simulink model "sampleModel1607_3_sub"  (R2023a)
settings: Solver=VariableStepAuto  StartTime=0.0  StopTime=10.0  RelTol=1e-3
libraries: hdlsllib x2, simulink x1
settings Model: Creator=user1  LastModifiedBy=user1

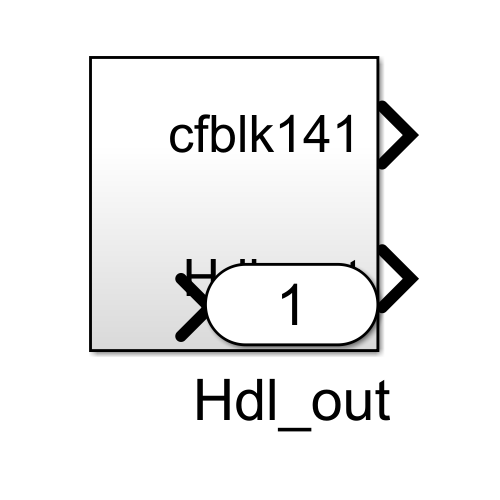
[thumbnail: Simulink's stored preview of the top-level diagram]
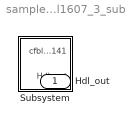
== system sampleModel1607_3_sub ==
  Subsystem : Subsystem
  Hdl_out : Outport  OutDataTypeStr=uint8

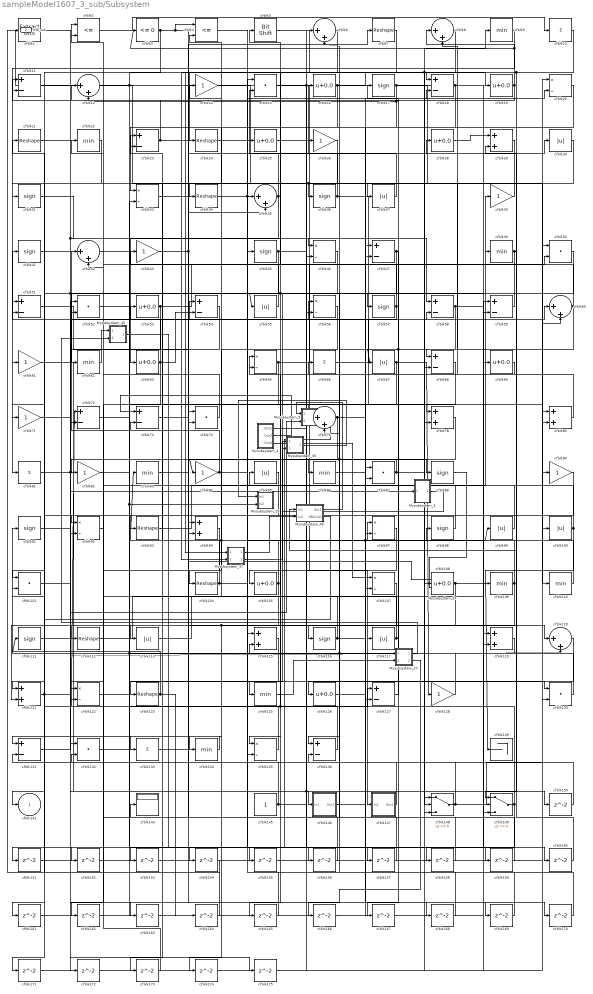
== system sampleModel1607_3_sub/Subsystem ==
  Mysubsystem_19 : Subsystem  TreatAsAtomicUnit=on  RTWFcnName=Mysubsystem_19
      settings: RTWFcnNameOpts=User specified  RTWFileNameOpts=Use function name
  Mysubsystem_2 : Subsystem  TreatAsAtomicUnit=on  RTWFcnName=Mysubsystem_2
      settings: RTWFcnNameOpts=User specified  RTWFileNameOpts=Use function name
  Mysubsystem_24 : Subsystem  TreatAsAtomicUnit=on  RTWFcnName=Mysubsystem_24
      settings: RTWFcnNameOpts=User specified  RTWFileNameOpts=Use function name
  Mysubsystem_27 : Subsystem  TreatAsAtomicUnit=on  RTWFcnName=Mysubsystem_27
      settings: RTWFcnNameOpts=User specified  RTWFileNameOpts=Use function name
  Mysubsystem_3 : Subsystem  TreatAsAtomicUnit=on  RTWFcnName=Mysubsystem_3
      settings: RTWFcnNameOpts=User specified  RTWFileNameOpts=Use function name
  Mysubsystem_35 : Subsystem  TreatAsAtomicUnit=on  RTWFcnName=Mysubsystem_35
      settings: RTWFcnNameOpts=User specified  RTWFileNameOpts=Use function name
  Mysubsystem_37 : Subsystem  TreatAsAtomicUnit=on  RTWFcnName=Mysubsystem_37
      settings: RTWFcnNameOpts=User specified  RTWFileNameOpts=Use function name
  Mysubsystem_43 : Subsystem  TreatAsAtomicUnit=on  RTWFcnName=Mysubsystem_43
      settings: RTWFcnNameOpts=User specified  RTWFileNameOpts=Use function name
  Mysubsystem_45 : Subsystem  TreatAsAtomicUnit=on  RTWFcnName=Mysubsystem_45
      settings: RTWFcnNameOpts=User specified  RTWFileNameOpts=Use function name
  Mysubsystem_5 : Subsystem  TreatAsAtomicUnit=on  RTWFcnName=Mysubsystem_5
      settings: RTWFcnNameOpts=User specified  RTWFileNameOpts=Use function name
  cfblk1 : simulink/Logic and Bit Operations/Extract Bits  bitsToExtract=Upper half  numBits=8  bitIdxRange=[0 7]  outScalingMode=Preserve fixed-point scaling
      settings: LibrarySourceBlock=|
      | hdlsllib/Logic and Bit
      | Operations/Extract Bits
  cfblk{10,66,81,133} (4 alike) : Sum  Inputs=+  OutDataTypeStr=uint8
  cfblk{30,37,55,67,85,99..100,113,117} (9 alike) : Abs  OutDataTypeStr=uint8  SaturateOnIntegerOverflow=off
  cfblk{15,50,52,74,87,101,130,132} (8 alike) : DotProduct  OutDataTypeStr=uint8
  cfblk{7,21,24,34,93,104,112,123} (8 alike) : Reshape
  cfblk{16,19,25,28,53,63,69,105,108,126} (10 alike) : Bias  Bias=0.0  SaturateOnIntegerOverflow=off
  cfblk{20,33,46,56,65,92,97,107,122,135} (10 alike) : Product  Inputs=*/  OutDataTypeStr=uint8  RndMeth=Zero  SaturateOnIntegerOverflow=on
  cfblk{9,22,49,62,83,86,109..110,125,134} (10 alike) : MinMax  OutDataTypeStr=uint8
  cfblk{11,18,23,47,51,54,58..59,68,72..73,127,131,136} (14 alike) : Sum  Inputs=+-  OutDataTypeStr=uint8
  cfblk{17,31,36,41,45,57,88,91,98,111,116} (11 alike) : Signum
  cfblk{29,78,80,94,115,119,121} (7 alike) : Sum  OutDataTypeStr=uint8
  cfblk{6,8,12,35,42,60,76,120} (8 alike) : Sum  Inputs=|++  OutDataTypeStr=uint8
  cfblk{14,26,39,43,61,71,82,84,90,128} (10 alike) : Gain  OutDataTypeStr=uint8
  cfblk139 : Terminator
  cfblk143 : Display
  cfblk145 : Constant  OutDataTypeStr=uint8  SampleTime=-1
  cfblk146 : Subsystem
      settings: LibrarySourceBlock=|
      | hdlsllib/Ports &
      | Subsystems/Subsystem
  cfblk147 : Subsystem
      settings: LibrarySourceBlock=|
      | hdlsllib/Ports &
      | Subsystems/Subsystem
  cfblk148 : Switch  OutDataTypeStr=uint8  SaturateOnIntegerOverflow=off  InputSameDT=off
  cfblk149 : Switch  OutDataTypeStr=uint8  SaturateOnIntegerOverflow=off  InputSameDT=off
  cfblk{150..175} (26 alike) : Delay  SampleTime=1
  cfblk2 : RelationalOperator  Operator=<=  OutDataTypeStr=boolean  InputSameDT=off
  cfblk3 : hdlsllib/Logic and Bit Operations/Compare To Zero  relop=<=  OutDataTypeStr=uint8
  cfblk4 : RelationalOperator  Operator=<=  OutDataTypeStr=boolean  InputSameDT=off
  cfblk5 : hdlsllib/Logic and Bit Operations/Bit Shift  mode=Shift Left Logical  N=0
  cfblk141 : Outport  OutDataTypeStr=uint8  VectorParamsAs1DForOutWhenUnconnected=off
  Hdl_out : Outport  Port=2  OutDataTypeStr=uint8
  wires:
  cfblk10/1 -> cfblk149/1, cfblk68/2, Mysubsystem_37/2(In2)
  cfblk9/1 -> cfblk81/1
  cfblk47/1 -> cfblk123/1, cfblk167/1, cfblk67/1
  cfblk35/1 -> cfblk15/2, cfblk63/1
  cfblk6/1 -> cfblk165/1, cfblk55/1
  cfblk61/1 -> cfblk146/1(In1)
  cfblk84/1 -> cfblk18/2, cfblk42/1
  cfblk2/1 -> cfblk10/1
  cfblk136/1 -> cfblk85/1, cfblk72/1
  cfblk120/1 -> cfblk143/1
  cfblk78/1 -> cfblk116/1, cfblk84/1
  cfblk108/1 -> cfblk121/2, cfblk139/1
  cfblk110/1 -> cfblk54/1, cfblk83/1
  cfblk24/1 -> cfblk100/1
  cfblk93/1 -> cfblk39/1
  cfblk97/1 -> cfblk135/1
  cfblk41/1 -> cfblk132/1
  cfblk67/1 -> cfblk125/1, cfblk128/1
  cfblk15/1 -> cfblk107/2, cfblk147/1(In1)
  cfblk99/1 -> cfblk65/1
  cfblk3/1 -> cfblk71/1, cfblk120/1, cfblk4/1
  cfblk31/1 -> cfblk46/1
  cfblk60/1 -> cfblk23/1, cfblk126/1
  cfblk107/1 -> cfblk174/1, cfblk133/1
  cfblk65/1 -> cfblk113/1, cfblk49/1
  cfblk26/1 -> cfblk93/1
  cfblk55/1 -> cfblk22/1
  cfblk149/1 -> cfblk171/1, cfblk66/1
  cfblk21/1 -> cfblk46/2
  cfblk22/1 -> cfblk61/1
  cfblk123/1 -> cfblk164/1, cfblk91/1
  cfblk36/1 -> cfblk25/1, cfblk110/1
  cfblk117/1 -> cfblk157/1, cfblk4/2
  cfblk39/1 -> cfblk31/1
  cfblk130/1 -> cfblk17/1
  cfblk57/1 -> cfblk51/2, cfblk5/1
  cfblk109/1 -> cfblk162/1, cfblk43/1
  cfblk104/1 -> cfblk98/1, cfblk73/2
  cfblk82/1 -> cfblk56/1
  cfblk49/1 -> cfblk117/1, Mysubsystem_43/1(In1)
  cfblk132/1 -> cfblk127/1
  cfblk20/1 -> cfblk105/1
  cfblk68/1 -> cfblk135/2
  cfblk98/1 -> cfblk2/1
  cfblk94/1 -> cfblk112/1
  cfblk8/1 -> cfblk24/1
  cfblk135/1 -> cfblk21/1
  cfblk134/1 -> cfblk131/1
  cfblk105/1 -> cfblk173/1, cfblk14/1
  cfblk119/1 -> cfblk115/2
  cfblk17/1 -> cfblk60/2, cfblk12/2, cfblk33/1
  cfblk37/1 -> cfblk16/1
  cfblk14/1 -> cfblk37/1
  cfblk126/1 -> cfblk20/2, cfblk99/1
  cfblk76/1 -> cfblk94/2, cfblk30/1
  cfblk127/1 -> cfblk97/1
  cfblk128/1 -> cfblk6/2, cfblk111/1
  cfblk28/1 -> cfblk29/1
  cfblk42/1 -> cfblk130/1, Mysubsystem_19/2(In2)
  cfblk116/1 -> cfblk149/3, cfblk2/2
  cfblk18/1 -> Hdl_out/1, cfblk87/2, cfblk119/1
  cfblk19/1 -> cfblk11/2, cfblk3/1, cfblk8/1
  cfblk63/1 -> cfblk54/2, cfblk92/1, cfblk41/1
  cfblk5/1 -> cfblk148/2
  cfblk121/1 -> cfblk151/1, cfblk150/1
  cfblk59/1 -> cfblk57/1
  cfblk80/1 -> cfblk8/2
  cfblk100/1 -> cfblk23/2, cfblk109/1
  cfblk16/1 -> cfblk19/1, cfblk34/1
  cfblk46/1 -> cfblk121/1
  cfblk72/1 -> cfblk78/1
  cfblk56/1 -> cfblk104/1
  cfblk33/1 -> cfblk35/2
  cfblk25/1 -> cfblk58/1
  cfblk147/1(Out1) -> cfblk51/1
  cfblk45/1 -> cfblk159/1, cfblk62/1
  cfblk131/1 -> cfblk52/1
  cfblk90/1 -> cfblk122/1
  cfblk51/1 -> cfblk74/2
  cfblk87/1 -> cfblk9/1, cfblk82/1
  cfblk122/1 -> Mysubsystem_27/1(In1), cfblk50/2
  cfblk1/1 -> cfblk120/2, cfblk59/2
  cfblk12/1 -> cfblk154/1, cfblk18/1, cfblk108/1
  cfblk113/1 -> cfblk45/1
  cfblk69/1 -> cfblk65/2
  cfblk85/1 -> cfblk101/1
  cfblk74/1 -> cfblk12/1
  cfblk58/1 -> cfblk160/1, cfblk76/1
  cfblk53/1 -> cfblk92/2, cfblk20/1
  cfblk50/1 -> cfblk136/1
  cfblk23/1 -> cfblk169/1, cfblk11/1
  cfblk11/1 -> cfblk168/1, cfblk47/2
  cfblk73/1 -> cfblk86/1
  cfblk112/1 -> cfblk69/1
  cfblk83/1 -> cfblk7/1
  cfblk115/1 -> cfblk134/1
  cfblk66/1 -> cfblk58/2
  cfblk81/1 -> cfblk53/1, Mysubsystem_3/1(In1)
  cfblk146/1(Out1) -> cfblk97/2
  cfblk52/1 -> cfblk80/2
  cfblk148/1 -> cfblk52/2, cfblk90/1
  cfblk34/1 -> cfblk26/1, cfblk88/1
  cfblk30/1 -> cfblk68/1
  cfblk133/1 -> cfblk94/1
  cfblk29/1 -> cfblk161/1, cfblk36/1
  cfblk43/1 -> cfblk28/1, Mysubsystem_24/1(In1)
  cfblk145/1 -> cfblk101/2, cfblk149/2, cfblk60/1
  cfblk150/1 -> cfblk132/2
  cfblk151/1 -> cfblk127/2
  cfblk92/1 -> cfblk152/1
  cfblk152/1 -> cfblk35/1
  cfblk54/1 -> cfblk153/1
  cfblk153/1 -> cfblk50/1
  cfblk154/1 -> cfblk1/1
  cfblk155/1 -> cfblk80/1
  cfblk4/1 -> cfblk156/1
  cfblk156/1 -> cfblk42/2
  cfblk157/1 -> cfblk122/2
  cfblk158/1 -> cfblk74/1
  cfblk159/1 -> cfblk76/2
  cfblk160/1 -> cfblk29/2
  cfblk161/1 -> cfblk78/2
  cfblk162/1 -> cfblk33/2
  cfblk91/1 -> cfblk163/1
  cfblk163/1 -> cfblk119/2
  cfblk164/1 -> cfblk131/2
  cfblk165/1 -> cfblk115/1
  cfblk166/1 -> cfblk47/1
  cfblk167/1 -> cfblk148/3
  cfblk168/1 -> cfblk15/1
  cfblk169/1 -> cfblk136/2
  cfblk86/1 -> cfblk170/1
  cfblk170/1 -> cfblk87/1
  cfblk171/1 -> cfblk56/2
  cfblk71/1 -> cfblk172/1
  cfblk172/1 -> cfblk59/1
  cfblk173/1 -> cfblk72/2
  cfblk174/1 -> cfblk130/2
  cfblk101/1 -> cfblk175/1
  cfblk175/1 -> cfblk148/1
  Mysubsystem_2/1(Out1) -> cfblk6/1
  Mysubsystem_2/2(Out2) -> cfblk73/1
  Mysubsystem_2/3(Out3) -> cfblk107/1
  cfblk111/1 -> Mysubsystem_5/2(In2)
  Mysubsystem_5/1(Out1) -> cfblk155/1
  cfblk88/1 -> Mysubsystem_24/2(In2)
  cfblk125/1 -> Mysubsystem_27/2(In2)
  Mysubsystem_27/2(Out2) -> cfblk166/1
  Mysubsystem_3/1(Out1) -> Mysubsystem_35/2(In2)
  Mysubsystem_35/1(Out1) -> Mysubsystem_19/1(In1)
  cfblk7/1 -> Mysubsystem_37/1(In1)
  Mysubsystem_37/2(Out2) -> Mysubsystem_35/1(In1)
  Mysubsystem_37/1(Out1) -> Mysubsystem_43/2(In2)
  Mysubsystem_43/1(Out1) -> Mysubsystem_5/1(In1)
  Mysubsystem_43/2(cfblk141) -> cfblk141/1
  cfblk62/1 -> Mysubsystem_45/1(In1)
  Mysubsystem_27/1(Out1) -> Mysubsystem_45/2(In2)
  Mysubsystem_45/1(Out1) -> cfblk158/1

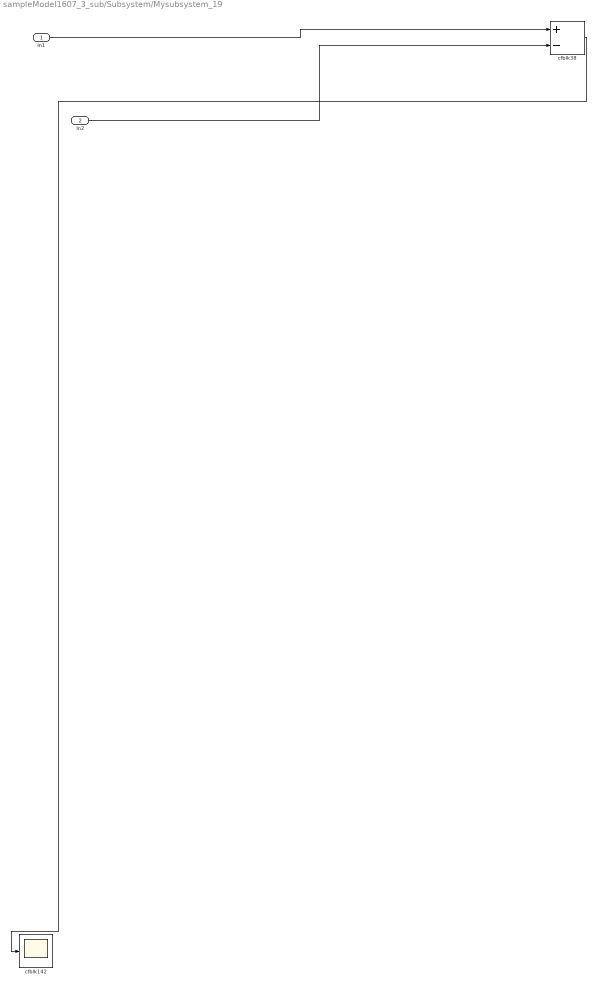
== system sampleModel1607_3_sub/Subsystem/Mysubsystem_19 ==
  In1 : Inport
  In2 : Inport  Port=2
  cfblk142 : Scope
  cfblk38 : Sum  Inputs=+-
  wires:
  In2/1 -> cfblk38/2
  In1/1 -> cfblk38/1
  cfblk38/1 -> cfblk142/1

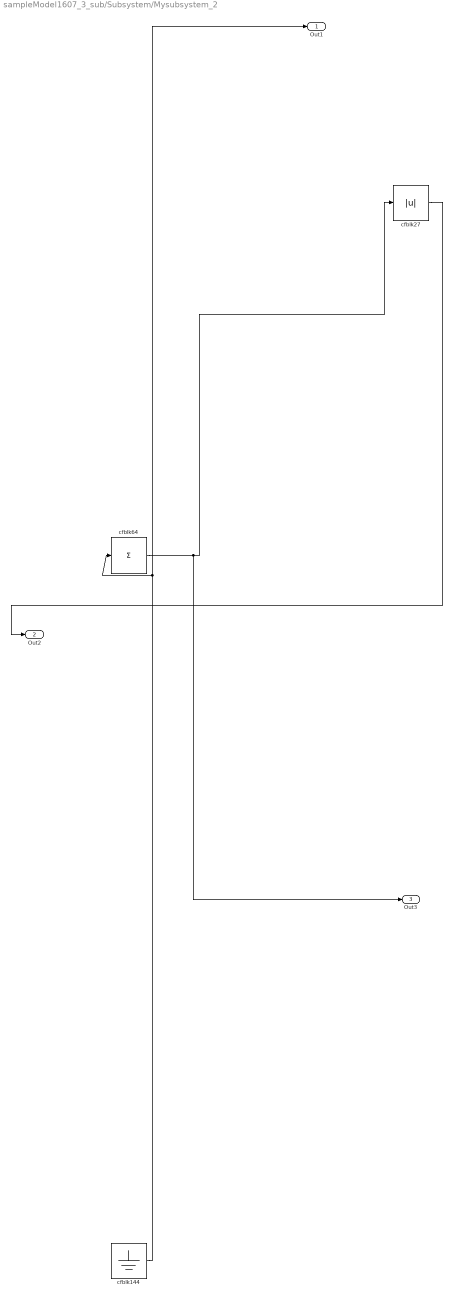
== system sampleModel1607_3_sub/Subsystem/Mysubsystem_2 ==
  cfblk144 : Ground
  cfblk27 : Abs  SaturateOnIntegerOverflow=off
  cfblk64 : Sum  Inputs=+
  Out1 : Outport
  Out2 : Outport  Port=2
  Out3 : Outport  Port=3
  wires:
  cfblk27/1 -> Out2/1
  cfblk144/1 -> cfblk64/1, Out1/1
  cfblk64/1 -> cfblk27/1, Out3/1

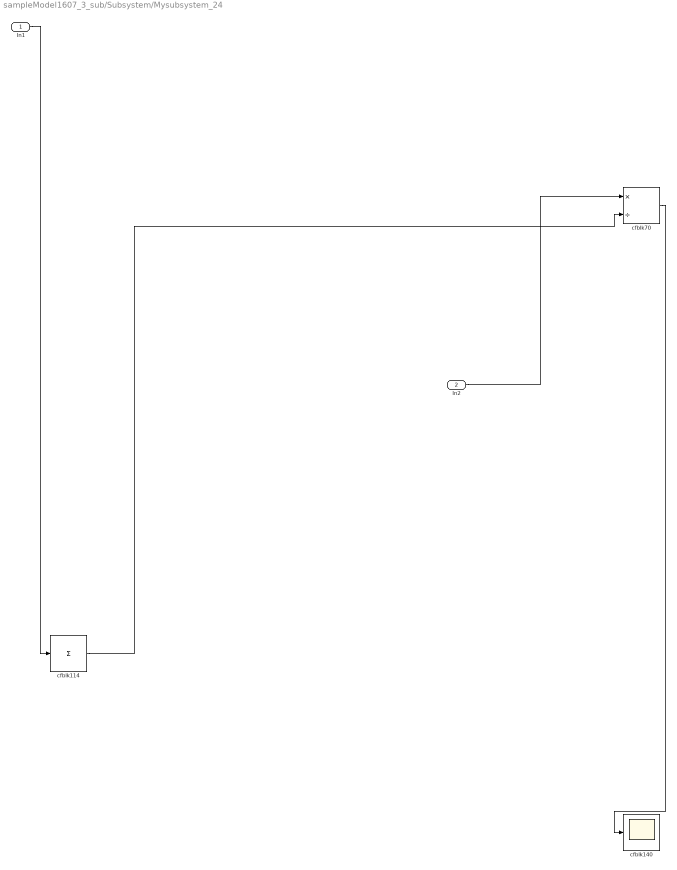
== system sampleModel1607_3_sub/Subsystem/Mysubsystem_24 ==
  In1 : Inport
  In2 : Inport  Port=2
  cfblk114 : Sum  Inputs=+
  cfblk140 : Scope
  cfblk70 : Product  Inputs=*/  RndMeth=Zero  SaturateOnIntegerOverflow=on
  wires:
  In1/1 -> cfblk114/1
  cfblk70/1 -> cfblk140/1
  cfblk114/1 -> cfblk70/2
  In2/1 -> cfblk70/1

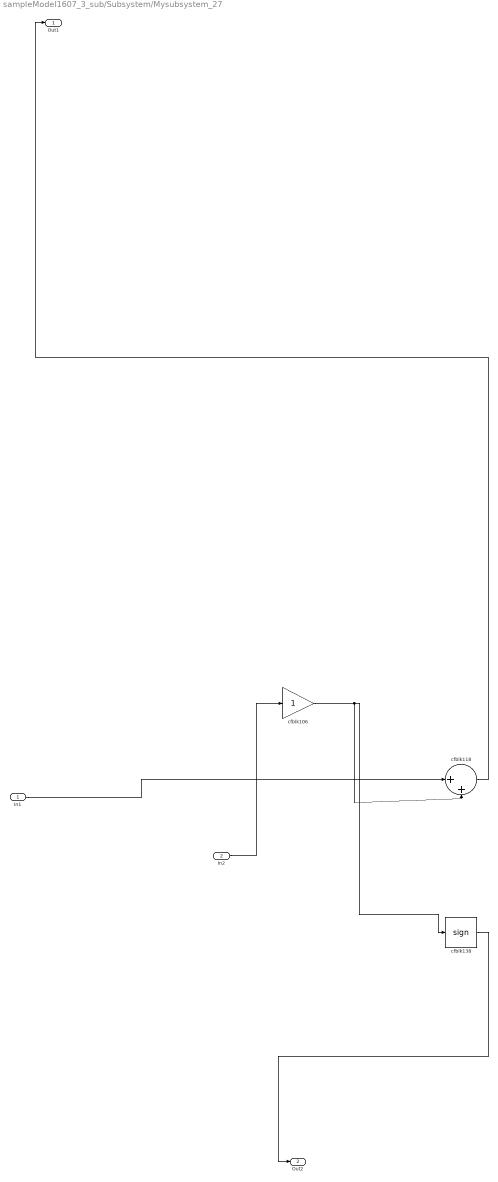
== system sampleModel1607_3_sub/Subsystem/Mysubsystem_27 ==
  In1 : Inport
  In2 : Inport  Port=2
  cfblk106 : Gain
  cfblk118 : Sum  Inputs=|++
  cfblk138 : Signum
  Out1 : Outport
  Out2 : Outport  Port=2
  wires:
  cfblk118/1 -> Out1/1
  In1/1 -> cfblk118/1
  cfblk138/1 -> Out2/1
  In2/1 -> cfblk106/1
  cfblk106/1 -> cfblk118/2, cfblk138/1

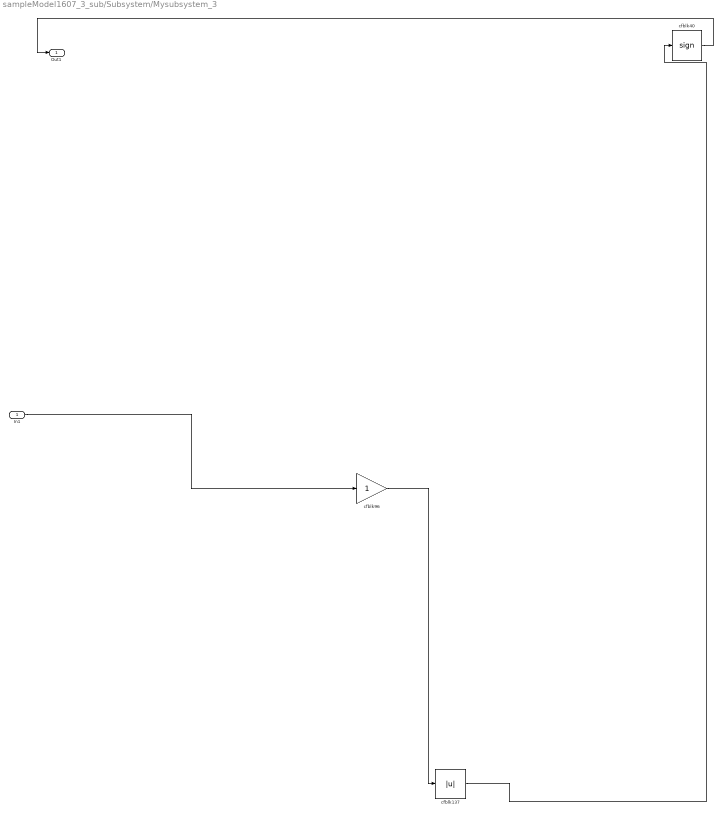
== system sampleModel1607_3_sub/Subsystem/Mysubsystem_3 ==
  In1 : Inport
  cfblk137 : Abs  SaturateOnIntegerOverflow=off
  cfblk40 : Signum
  cfblk96 : Gain
  Out1 : Outport
  wires:
  cfblk40/1 -> Out1/1
  cfblk137/1 -> cfblk40/1
  In1/1 -> cfblk96/1
  cfblk96/1 -> cfblk137/1

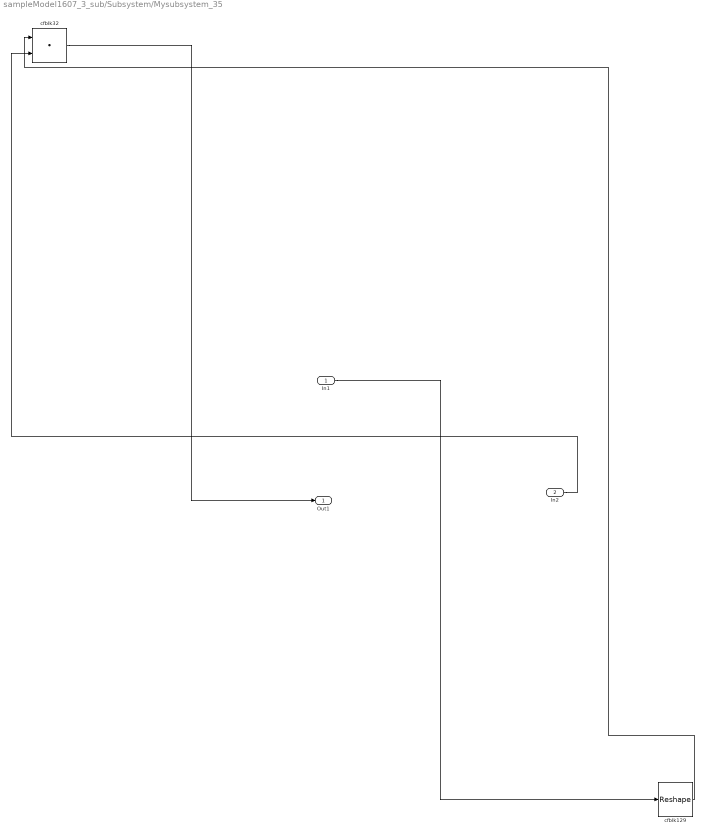
== system sampleModel1607_3_sub/Subsystem/Mysubsystem_35 ==
  In1 : Inport
  In2 : Inport  Port=2
  cfblk129 : Reshape
  cfblk32 : DotProduct  OutDataTypeStr=Inherit: Inherit via internal rule
  Out1 : Outport
  wires:
  In1/1 -> cfblk129/1
  In2/1 -> cfblk32/2
  cfblk32/1 -> Out1/1
  cfblk129/1 -> cfblk32/1

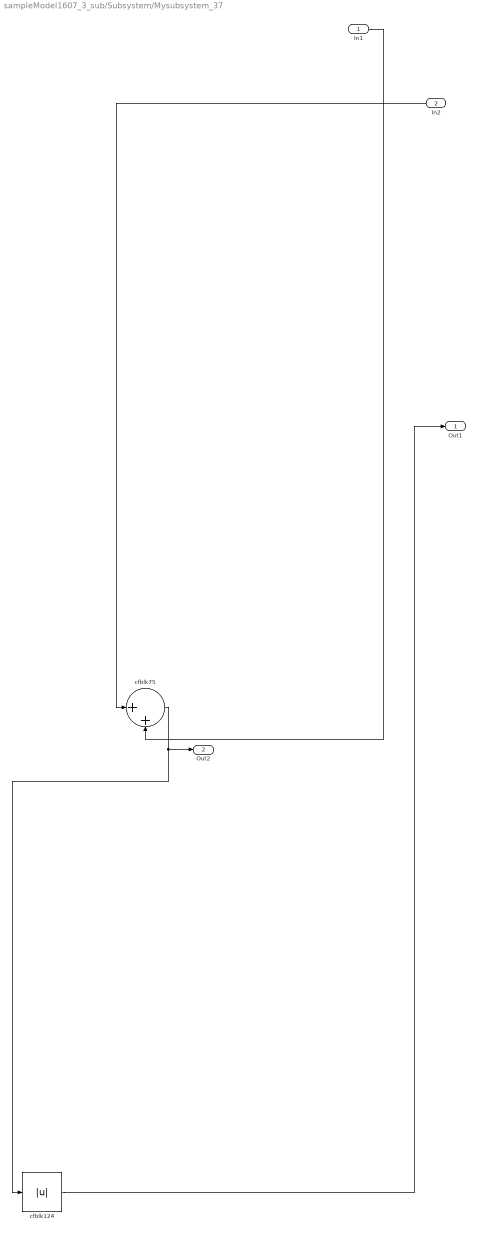
== system sampleModel1607_3_sub/Subsystem/Mysubsystem_37 ==
  In1 : Inport
  In2 : Inport  Port=2
  cfblk124 : Abs  SaturateOnIntegerOverflow=off
  cfblk75 : Sum  Inputs=|++
  Out1 : Outport
  Out2 : Outport  Port=2
  wires:
  cfblk124/1 -> Out1/1
  In2/1 -> cfblk75/1
  In1/1 -> cfblk75/2
  cfblk75/1 -> cfblk124/1, Out2/1

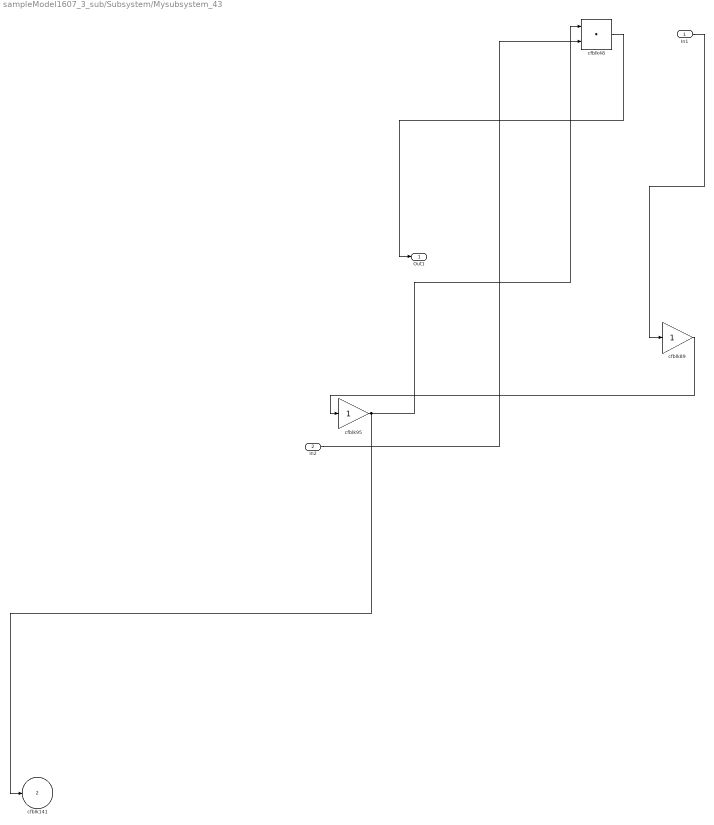
== system sampleModel1607_3_sub/Subsystem/Mysubsystem_43 ==
  In1 : Inport
  In2 : Inport  Port=2
  cfblk48 : DotProduct  OutDataTypeStr=Inherit: Inherit via internal rule
  cfblk89 : Gain
  cfblk95 : Gain
  Out1 : Outport
  cfblk141 : Outport  Port=2  VectorParamsAs1DForOutWhenUnconnected=off
  wires:
  In2/1 -> cfblk48/2
  cfblk48/1 -> Out1/1
  In1/1 -> cfblk89/1
  cfblk95/1 -> cfblk48/1, cfblk141/1
  cfblk89/1 -> cfblk95/1

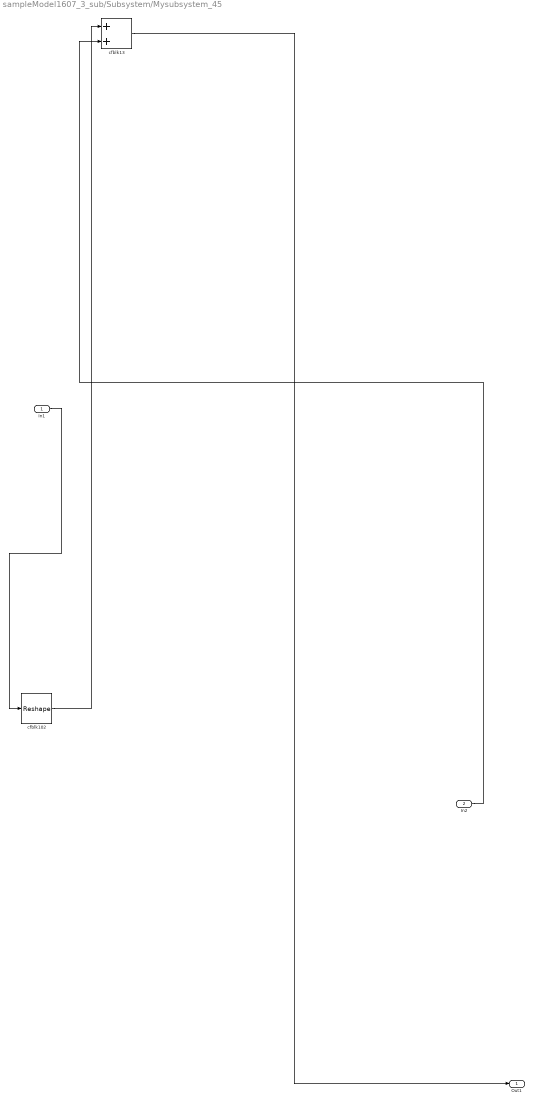
== system sampleModel1607_3_sub/Subsystem/Mysubsystem_45 ==
  In1 : Inport
  In2 : Inport  Port=2
  cfblk102 : Reshape
  cfblk13 : Sum
  Out1 : Outport
  wires:
  cfblk13/1 -> Out1/1
  In1/1 -> cfblk102/1
  In2/1 -> cfblk13/2
  cfblk102/1 -> cfblk13/1

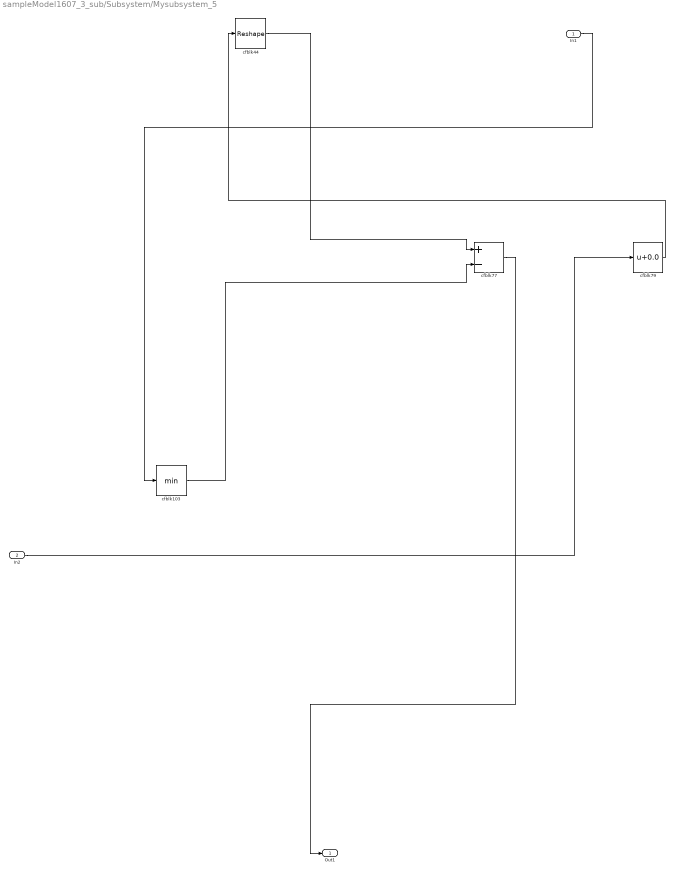
== system sampleModel1607_3_sub/Subsystem/Mysubsystem_5 ==
  In1 : Inport
  In2 : Inport  Port=2
  cfblk103 : MinMax
  cfblk44 : Reshape
  cfblk77 : Sum  Inputs=+-
  cfblk79 : Bias  Bias=0.0  SaturateOnIntegerOverflow=off
  Out1 : Outport
  wires:
  cfblk77/1 -> Out1/1
  In1/1 -> cfblk103/1
  In2/1 -> cfblk79/1
  cfblk79/1 -> cfblk44/1
  cfblk103/1 -> cfblk77/2
  cfblk44/1 -> cfblk77/1

== system sampleModel1607_3_sub/Subsystem/cfblk146 ==
  In1 : Inport
  Out1 : Outport
  wires:
  In1/1 -> Out1/1

== system sampleModel1607_3_sub/Subsystem/cfblk147 ==
  In1 : Inport
  Out1 : Outport
  wires:
  In1/1 -> Out1/1
